simulink subsystem "RT_FlappingDynamic_v1_2"  (R2025a)
settings: Solver=VariableStepAuto  StartTime=0.0  StopTime=10.0  RelTol=1e-3
model mask{RT_BEDistFromEffSta=RT_BEDistFromEffSta, RT_RotorRadius=RT_RotorRadius, RT_BladeFlapInertia=RT_BladeFlapInertia, RT_BEMassFromHinge=RT_BEMassFromHinge, RT_BEDistFromHinge=RT_BEDistFromHinge, RT_HingeFlapPos=RT_HingeFlapPos}
  mask prompts: RT_BEDistFromEffSta "Distance from effective station to blade element [-]"; RT_RotorRadius "Rotor radius [m]"; RT_BladeFlapInertia "Blade flapping moment of inertia [kg·m²]"; RT_BEMassFromHinge "Blade element mass from flapping hinge [kg]"; RT_BEDistFromHinge "Distance from flapping hinge to blade element [-]"; RT_HingeFlapPos "Flapping hinge position [-]"
settings Model: DefaultTestHarness=RT_FlappingDynamic_v1_1_Harness1  Creator=ADMIN  LastModifiedBy=Admin

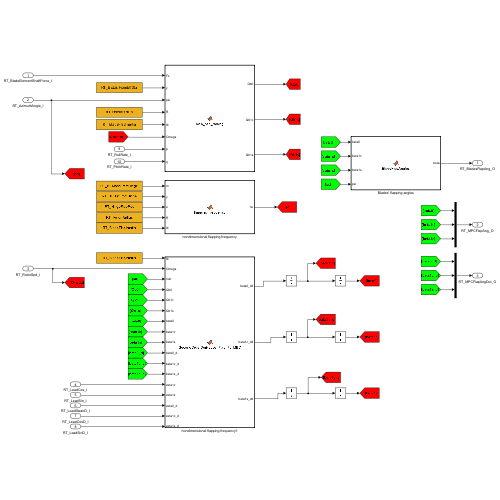
[thumbnail: Simulink's stored preview of the top-level diagram]
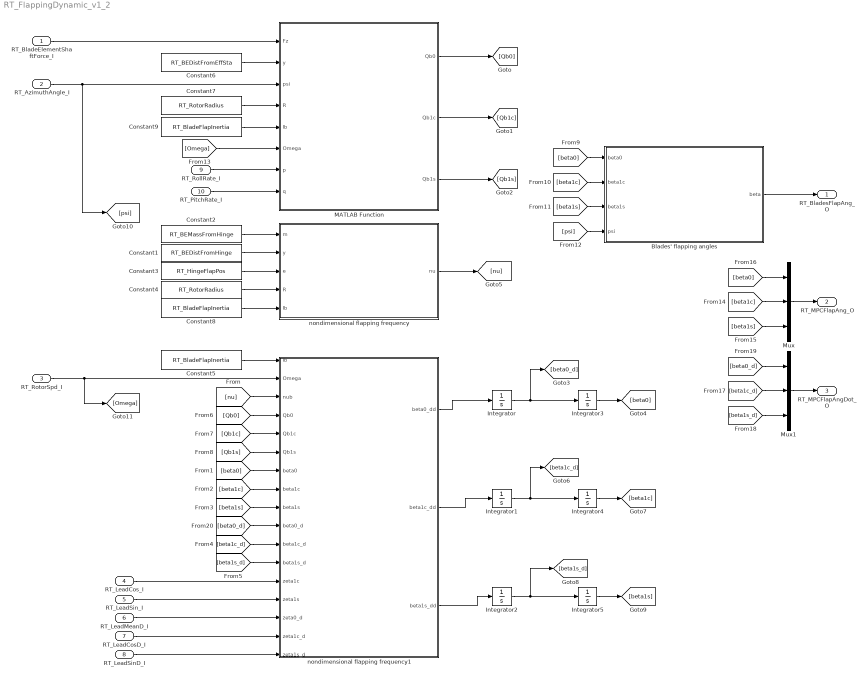
== system RT_FlappingDynamic_v1_2 ==
  RT_BladeElementShaftForce_I : Inport
  RT_AzimuthAngle_I : Inport  Port=2
  RT_RotorSpd_I : Inport  Port=3
  RT_LeadCos_I : Inport  Port=4
  RT_LeadSin_I : Inport  Port=5
  RT_LeadMeanD_I : Inport  Port=6
  RT_LeadCosD_I : Inport  Port=7
  RT_LeadSinD_I : Inport  Port=8
  RT_RollRate_I : Inport  Port=9
  RT_PitchRate_I : Inport  Port=10
  Blades' flapping angles : MATLAB Function  TreatAsAtomicUnit=on
  Constant1 : Constant  Value=RT_BEDistFromHinge
  Constant2 : Constant  Value=RT_BEMassFromHinge
  Constant3 : Constant  Value=RT_HingeFlapPos
  Constant4 : Constant  Value=RT_RotorRadius
  Constant5 : Constant  Value=RT_BladeFlapInertia
  Constant6 : Constant  Value=RT_BEDistFromEffSta
  Constant7 : Constant  Value=RT_RotorRadius
  Constant8 : Constant  Value=RT_BladeFlapInertia
  Constant9 : Constant  Value=RT_BladeFlapInertia
  Integrator{,1..5} (6 alike) : Integrator
  MATLAB Function : MATLAB Function  TreatAsAtomicUnit=on
  Mux : Mux  Inputs=3
  Mux1 : Mux  Inputs=3
  nondimensional flapping frequency : MATLAB Function  TreatAsAtomicUnit=on
  nondimensional flapping frequency1 : MATLAB Function  TreatAsAtomicUnit=on
  RT_BladesFlapAng_O : Outport
  RT_MPCFlapAng_O : Outport  Port=2
  RT_MPCFlapAngDot_O : Outport  Port=3
  wires:
  nondimensional flapping frequency1/2(beta1c_dd) -> Integrator1/1
  [beta1c] -> Blades' flapping angles/2(beta1c)
  RT_LeadCos_I/1 -> nondimensional flapping frequency1/13(zeta1c)
  Integrator3/1 -> [beta0]
  MATLAB Function/3(Qb1s) -> [Qb1s]
  Integrator2/1 -> [beta1s_d], Integrator5/1
  Constant1/1 -> nondimensional flapping frequency/2(y)
  Constant2/1 -> nondimensional flapping frequency/1(m)
  [psi] -> Blades' flapping angles/4(psi)
  Integrator5/1 -> [beta1s]
  Constant7/1 -> MATLAB Function/4(R)
  [beta1s_d] -> Mux1/3
  [Qb1s] -> nondimensional flapping frequency1/6(Qb1s)
  RT_BladeElementShaftForce_I/1 -> MATLAB Function/1(Fz)
  Integrator/1 -> [beta0_d], Integrator3/1
  Constant9/1 -> MATLAB Function/5(Ib)
  [beta1c] -> nondimensional flapping frequency1/8(beta1c)
  Mux1/1 -> RT_MPCFlapAngDot_O/1
  Mux/1 -> RT_MPCFlapAng_O/1
  [beta1c_d] -> nondimensional flapping frequency1/11(beta1c_d)
  RT_LeadSinD_I/1 -> nondimensional flapping frequency1/17(zeta1s_d)
  RT_LeadCosD_I/1 -> nondimensional flapping frequency1/16(zeta1c_d)
  RT_LeadMeanD_I/1 -> nondimensional flapping frequency1/15(zeta0_d)
  [beta0] -> Blades' flapping angles/1(beta0)
  RT_PitchRate_I/1 -> MATLAB Function/8(q)
  [beta1c_d] -> Mux1/2
  Blades' flapping angles/1(beta) -> RT_BladesFlapAng_O/1
  [beta1s] -> Mux/3
  nondimensional flapping frequency1/3(beta1s_dd) -> Integrator2/1
  [beta0] -> nondimensional flapping frequency1/7(beta0)
  [Omega] -> MATLAB Function/6(Omega)
  RT_RollRate_I/1 -> MATLAB Function/7(p)
  [beta1s_d] -> nondimensional flapping frequency1/12(beta1s_d)
  [beta1c] -> Mux/2
  Integrator1/1 -> [beta1c_d], Integrator4/1
  [nu] -> nondimensional flapping frequency1/3(nub)
  Constant6/1 -> MATLAB Function/2(y)
  Constant5/1 -> nondimensional flapping frequency1/1(Ib)
  [Qb1c] -> nondimensional flapping frequency1/5(Qb1c)
  Constant4/1 -> nondimensional flapping frequency/4(R)
  nondimensional flapping frequency1/1(beta0_dd) -> Integrator/1
  RT_RotorSpd_I/1 -> [Omega], nondimensional flapping frequency1/2(Omega)
  [beta1s] -> nondimensional flapping frequency1/9(beta1s)
  Constant8/1 -> nondimensional flapping frequency/5(Ib)
  RT_AzimuthAngle_I/1 -> [psi], MATLAB Function/3(psi)
  [beta0_d] -> Mux1/1
  MATLAB Function/1(Qb0) -> [Qb0]
  RT_LeadSin_I/1 -> nondimensional flapping frequency1/14(zeta1s)
  [beta1s] -> Blades' flapping angles/3(beta1s)
  Integrator4/1 -> [beta1c]
  nondimensional flapping frequency/1(nu) -> [nu]
  MATLAB Function/2(Qb1c) -> [Qb1c]
  Constant3/1 -> nondimensional flapping frequency/3(e)
  [beta0] -> Mux/1
  [Qb0] -> nondimensional flapping frequency1/4(Qb0)
  [beta0_d] -> nondimensional flapping frequency1/10(beta0_d)

== matlab function RT_FlappingDynamic_v1_2/nondimensional flapping frequency ==
  data: m input; nu output; y input; e input; R input; Ib input
function nu  = flapping_frequency(m, y, e, R, Ib)
% m   : [1 x Ns] radial element mass from hinge (kg)
% y   : [1 x Ns]  radial stations from hinge (m)  
% e   : [1 x 1]  hinge ratio with radius (-)
% R   : [1 x 1]  Radius of rotor blade
% Ib  :
% Returns blade flapping natural frequency (N·m)

      
    nu = 1 + e*R/Ib*(m'*y);
end

== matlab function RT_FlappingDynamic_v1_2/nondimensional flapping frequency1 ==
  data: Ib input; Omega input; nub input; Qb0 input; beta0_dd output; Qb1c input; Qb1s input; beta0 input; beta1c input; beta1s input; beta0_d input; beta1c_d input; beta1s_d input; zeta1c input; zeta1s input; zeta0_d input; beta1c_dd output; beta1s_dd output; zeta1c_d input; zeta1s_d input
function [beta0_dd, beta1c_dd, beta1s_dd] = SecondOrderDerivative_Flap_FullMBC( ...
    Ib, Omega, nub, ...
    Qb0, Qb1c, Qb1s, ...
    beta0, beta1c, beta1s, ...
    beta0_d, beta1c_d, beta1s_d, ...
    zeta1c, zeta1s, ...
    zeta0_d, zeta1c_d, zeta1s_d)
%#codegen
% Full MBC flap dynamics with Coriolis coupling + structural damping
% 
% Signs:
%   Gyroscopic: -2*Omega*beta1s_d in beta1c, +2*Omega*beta1c_d in beta1s
%   Coriolis:   +2*Omega (flap)
%   Damping:    cross-coupled via (rate + Omega*position) structure
%
% nub = nu_beta^2 (squared flap frequency)

% === Structural / numerical flap damping (per-blade, rotating frame) ===
% Note: Aerodynamic damping (Lock number effect) is already in Qb forcing
%       if BET computes UP with beta_d*r term correctly.
%       C_beta here is for numerical stabilization only.
    C_beta = 100.0;   % N·m·s/rad (tune for numerical stability)

% === MBC damping terms ===
    Db0  = C_beta * beta0_d;
    Db1c = C_beta * (beta1c_d + Omega * beta1s);
    Db1s = C_beta * (beta1s_d - Omega * beta1c);

% === Coriolis projections (sign = +2*Omega for flap) ===
    P0 = beta0 * zeta0_d ...
       + 0.5 * (beta1c * zeta1c_d + beta1s * zeta1s_d) ...
       + 0.5 * Omega * (beta1c * zeta1s - beta1s * zeta1c);

    P1c = beta0 * zeta1c_d ...
        + Omega * beta0 * zeta1s ...
        + beta1c * zeta0_d;

    P1s = beta0 * zeta1s_d ...
        - Omega * beta0 * zeta1c ...
        + beta1s * zeta0_d;

% === Coning flap ===
    beta0_dd = (Qb0 - Db0)/Ib ...
             - nub * Omega^2 * beta0 ...
             + 2 * Omega * P0;

% === Longitudinal cyclic flap ===
    beta1c_dd = (Qb1c - Db1c)/Ib ...
              - 2 * Omega * beta1s_d ...
              - (nub - 1) * Omega^2 * beta1c ...
              + 2 * Omega * P1c;

% === Lateral cyclic flap ===
    beta1s_dd = (Qb1s - Db1s)/Ib ...
              + 2 * Omega * beta1c_d ...
              - (nub - 1) * Omega^2 * beta1s ...
              + 2 * Omega * P1s;
end

== matlab function RT_FlappingDynamic_v1_2/Blades' flapping angles ==
  data: beta0 input; beta output; beta1c input; beta1s input; psi input
function beta   = BladeFlapAngles(beta0, beta1c, beta1s, psi)
    
    beta = beta0 + beta1c*cos(psi) + beta1s*sin(psi);
end

== matlab function RT_FlappingDynamic_v1_2/MATLAB Function ==
  data: Fz input; Qb0 output; y input; psi input; Qb1c output; R input; Qb1s output; Ib input; Omega input; p input; q input
function [Qb0, Qb1c, Qb1s] = mbc_flap_forcing(Fz, y, psi, R, Ib, Omega, p, q)
    % MBC flap forcing - COMPILER SAFE VERSION
    
    psi = psi(:);
    y = y(:);
    Nb = length(psi); 
    Ns = length(y);   
    
    Qa = zeros(Nb, 1);
    
    % Khởi tạo cứng ma trận 4x20
    Fz_correct = zeros(Nb, Ns);
    
    % LƯỚI LỌC COMPILER: Chỉ reshape nếu số lượng phần tử thực sự là 80 (Nb * Ns)
    if numel(Fz) == (Nb * Ns)
        if size(Fz, 1) == Ns && size(Fz, 2) == Nb
            Fz_correct = Fz'; % Đảo từ [20x4] thành [4x20]
        elseif size(Fz, 1) == Nb && size(Fz, 2) == Ns
            Fz_correct = Fz;  % Chuẩn [4x20]
        else
            Fz_correct = reshape(Fz, [Nb, Ns]); % Ép mảng 1D thành [4x20]
        end
    else
        % Nếu Compiler đưa vào 1x1, gán tạm giá trị đó cho toàn bộ 80 ô để vượt rào
        Fz_correct(:, :) = Fz(1); 
    end
    
    % Tính Moment
    for b = 1:Nb
        moment_sum = 0;
        for i = 1:Ns
            moment_sum = moment_sum + Fz_correct(b, i) * y(i) * R;
        end
        Qa(b) = moment_sum;
    end
    
    Qa0  = sum(Qa) / Nb;
    Qa1c = (2 / Nb) * sum(Qa .* cos(psi));
    Qa1s = (2 / Nb) * sum(Qa .* sin(psi));
    
    Qg0  = 0;
    Qg1c = -2 * Ib * Omega * p;
    Qg1s = -2 * Ib * Omega * q;
    
    Qb0  = Qa0  + Qg0;
    Qb1c = Qa1c + Qg1c;
    Qb1s = Qa1s + Qg1s;
end
